simulink model "SimDraft1"  (R2024a)
settings: Solver=VariableStepAuto  StartTime=0.0  StopTime=2  RelTol=1e-3
model workspace (MAT data in the model file):
  CanaryCarrierFrequency = 20000
  CanaryDataRate = 100
  SampleRate = 44100
undefined symbols (not defined in the file or in its folder): azelaxes, fdesignblkfcn, gcbh, physconst
libraries: audiosources x2, dspfdesign x2, commseqgen3 x2, dspfiltersrcs x1, dspmlti4 x1, commanapbnd3 x1, dsparch4 x1, commdigbbndam3 x1, phasedenvlib x1
settings Model: Creator=calum  LastModifiedBy=calum

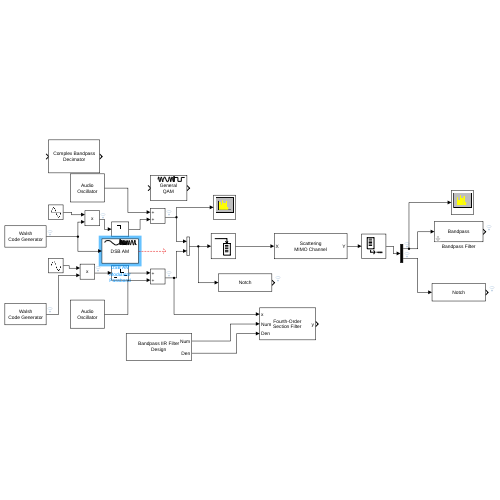
[thumbnail: Simulink's stored preview of the top-level diagram]
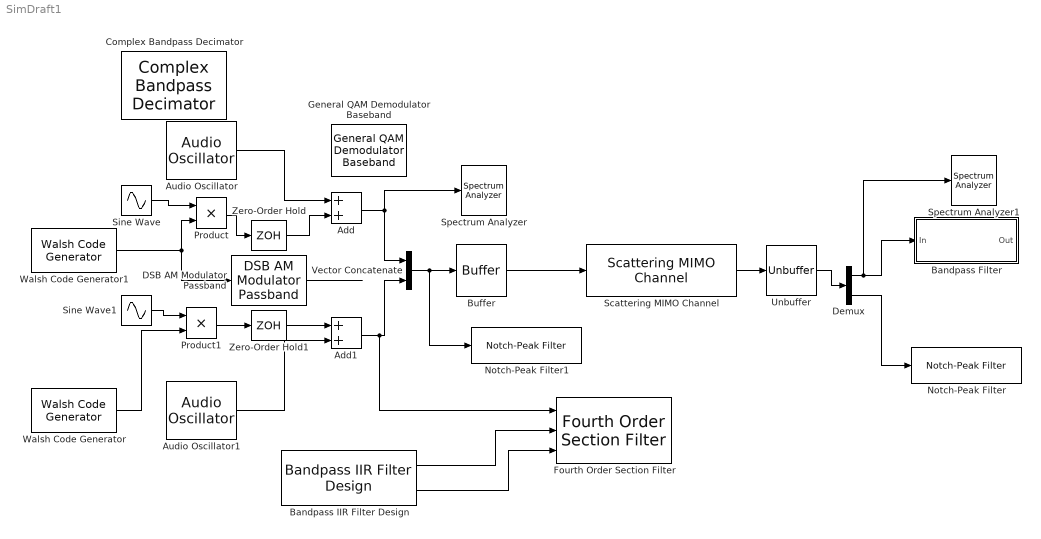
== system SimDraft1 ==
  Add : Sum
  Add1 : Sum
  Audio Oscillator : audiosources/Audio Oscillator  FrequencyPort=off  Frequency=200  AmplitudePort=off  Amplitude=1  DCOffsetPort=off  DCOffset=0  PhaseOffset=0  WidthPort=off  Width=1  DutyCyclePort=off  DutyCycle=0.5  SampsPerFrame=1  Fs=SampleRate  OutputDataType=double  SimulateUsing=Code generation
      settings: SignalType=sine
  Audio Oscillator1 : audiosources/Audio Oscillator  FrequencyPort=off  Frequency=500  AmplitudePort=off  Amplitude=1  DCOffsetPort=off  DCOffset=0  PhaseOffset=0  WidthPort=off  Width=1  DutyCyclePort=off  DutyCycle=0.5  SampsPerFrame=1  Fs=SampleRate  OutputDataType=double  SimulateUsing=Code generation
      settings: SignalType=sine
  Bandpass Filter : Subsystem  DialogController=fdesignblkfcn  InitFcn=fdesignblkfcn(gcbh, {'InitFcn'});  mask(Bandpass Filter){}
      mask help: dsp:DSPFilterDesignBlockDialog:BandpassFdesign_MaskDesc
      settings: CopyFcn=fdesignblkfcn(gcbh, {'CopyFcn'});
      mask Help: helpview(mapfilelocation('dsp'), 'dspbandpassfilter');
      mask Display: disp('Bandpass');
  Bandpass IIR Filter Design : dspfiltersrcs/Bandpass IIR Filter Design  SmoothParameters=off  SmoothingFactor=0.6  DesignMethod=Butterworth  FilterOrderPort=off  FilterOrder=6  MaxOrder=10  F3dB1Port=off  F3dB1=(CanaryCarrierFrequency-CanaryDataRate)/SampleRate/2  F3dB2Port=off  F3dB2=(CanaryCarrierFrequency+CanaryDataRate)/SampleRate/2  ApassPort=off  Apass=1  AstopPort=off  Astop=60  CascadeSectionsForm=Fourth-order sections  HasScaleValues=off  OutputDataType=double  SampleTime=-1  SimulateUsing=Interpreted execution
  Buffer : Buffer  OutputFrames=off
  Complex Bandpass Decimator : dspmlti4/Complex Bandpass Decimator  Specification=Bandwidth  DecimationFactor=2  Bandwidth=CanaryDataRate  CenterFrequencyPort=off  CenterFrequency=CanaryCarrierFrequency  StopbandAttenuation=80  PassbandRipple=1  TransitionWidth=40  MinimizeComplexCoefficients=on  MixToBaseband=on  InheritSampleRate=off  SampleRate=SampleRate  AllowArbitraryInputLength=off  SimulateUsing=Interpreted execution
  DSB AM Modulator Passband : commanapbnd3/DSB AM Modulator Passband  Fc=CanaryCarrierFrequency  Ph=0  Offset=1
  Demux : Demux  Outputs=2
  Fourth Order Section Filter : dsparch4/Fourth Order Section Filter  CoefficientSource=Input ports  Numerator=[0.07795634 0 -0.15591268 0 0.07795634; 0.06188520 0 -0.12377039 0 0.06188520]  Denominator=[1 0 1.32091343 0 0.63273879; 1 0 1.04859957 0 0.29614035]  FilterObject=dsp.FourthOrderSectionFilter  SimulateUsing=Code generation
  General QAM Demodulator Baseband : commdigbbndam3/General QAM Demodulator Baseband  SigCon=[exp(2*pi*1i*[0:7]/8)]  OutType=Integer  DecType=Hard decision  VarSource=Dialog  Variance=1  outDtypeBit=Inherit via internal rule  outDtype=Inherit via internal rule  roundingMode=Floor  overflowMode=Wrap  OvFlMode=off  OvFlModeLastStrValue=off  sigConstWordLen=16  sigConstDataTypeStr=Inherit: Same word length as input  sigConstLastDataTypeStr=Inherit: Same word length as input  accum1WordLen=32  accum1FracLen=30  prodInWordLen=32  prodInFracLen=30  prodInDataTypeStr=Inherit: Same as accumulator 1  prodInLastDataTypeStr=Inherit: Same as accumulator 1  prodOutWordLen=32  prodOutFracLen=30  accum2WordLen=32  accum2FracLen=30  accum3WordLen=32  accum3FracLen=30  nsiWordLen=32  nsiFracLen=30  nsiDataTypeStr=Inherit: Same as accumulator 3  nsiLastDataTypeStr=Inherit: Same as accumulator 3  invn0WordLen=16  invn0FracLen=8  invn0DataTypeStr=Inherit: Same word length as input  invn0LastDataTypeStr=Inherit: Same word length as input  outputWordLen=32  outputFracLen=30
  Notch-Peak Filter : dspfdesign/Notch-Peak Filter  Specification=Bandwidth and center frequency  BandwidthPort=off  Bandwidth=200  QualityFactorPort=off  QualityFactor=5  CenterFrequencyPort=off  CenterFrequency=20000  BandwidthCoefficientPort=off  BandwidthCoefficient=0.72654  CenterFrequencyCoefficientPort=off  CenterFrequencyCoefficient=0  Output=Notch  SampleRateMode=Specify on dialog  SampleRate=44100  SimulateUsing=Code generation
  Notch-Peak Filter1 : dspfdesign/Notch-Peak Filter  Specification=Bandwidth and center frequency  BandwidthPort=off  Bandwidth=200  QualityFactorPort=off  QualityFactor=5  CenterFrequencyPort=off  CenterFrequency=CanaryCarrierFrequency  BandwidthCoefficientPort=off  BandwidthCoefficient=0.72654  CenterFrequencyCoefficientPort=off  CenterFrequencyCoefficient=0  Output=Notch  SampleRateMode=Specify on dialog  SampleRate=SampleRate  SimulateUsing=Code generation
  Product : Product
  Product1 : Product
  Scattering MIMO Channel : phasedenvlib/Scattering MIMO Channel  PropagationSpeed=300  CarrierFrequency=CanaryCarrierFrequency  Polarization=None  SpecifyAtmosphere=off  Temperature=15  DryAirPressure=101325  WaterVapourDensity=7.5  LiquidWaterDensity=0  RainRate=0  SampleRateFromInputCheckbox=on  SampleRate=1e6  SimulateDirectPath=on  MaximumDelaySource=Property  MaximumDelay=2  ChannelResponseOutputPort=off  SimulateUsing=Code generation  TransmitArray=phased.ULA(Element=phased.OmnidirectionalMicrophoneElement())  ReceiveArray=phased.ULA(Element=phased.OmnidirectionalMicrophoneElement())  TransmitArrayMotionSource=Property  TransmitArrayPosition=[ 0; 0; 0 ]  TransmitArrayOrientationAxes=eye( 3 )  ReceiveArrayMotionSource=Property  ReceiveArrayPosition=[ 10; 0; 0 ]  ReceiveArrayOrientationAxes=azelaxes( 180, 0 )  ScattererSpecificationSource=Auto  NumScatterers=0  ScattererPositionBoundary=[ 0, 1000 ]  ScattererPosition=[ physconst( 'LightSpeed' )*5e-6; 0; 0 ]  ScattererCoefficient=1  ScatteringMatrix=eye( 2 )  ScattererOrientationAxes=eye( 3 )  SeedSource=Auto  Seed=0
  Sine Wave : Sin  Frequency=2*pi*CanaryCarrierFrequency  SampleTime=0
  Sine Wave1 : Sin  Frequency=2*pi*CanaryCarrierFrequency  SampleTime=0
  Spectrum Analyzer : SpectrumAnalyzer  SampleRateSource=Property  SampleRate=44.1e3  PlotAsTwoSidedSpectrum=off  FrequencyScale=Log  FrequencySpan=Start and stop frequencies  StartFrequency=20  StopFrequency=20e3
  Spectrum Analyzer1 : SpectrumAnalyzer  SampleRateSource=Property  SampleRate=44.1e3  PlotAsTwoSidedSpectrum=off  FrequencyScale=Log  FrequencySpan=Start and stop frequencies  StartFrequency=20  StopFrequency=20e3
  Unbuffer : Unbuffer
  Vector Concatenate : Concatenate  Mode=Multidimensional array  ConcatenateDimension=2
  Walsh Code Generator : commseqgen3/Walsh Code Generator  Length=16  Index=8  SampleTime=1/CanaryDataRate  SamplesPerFrame=1  OutputDataType=double  SimulateUsing=Code generation
  Walsh Code Generator1 : commseqgen3/Walsh Code Generator  Length=16  Index=8  SampleTime=1/CanaryDataRate  SamplesPerFrame=1  OutputDataType=double  SimulateUsing=Code generation
  Zero-Order Hold : ZeroOrderHold  SampleTime=1/SampleRate
  Zero-Order Hold1 : ZeroOrderHold  SampleTime=1/SampleRate
  wires:
  Vector Concatenate/1 -> Notch-Peak Filter1/1, Buffer/1
  Sine Wave/1 -> Product/1
  Sine Wave1/1 -> Product1/1
  Walsh Code Generator/1 -> Product1/2
  Product/1 -> Zero-Order Hold/1
  Audio Oscillator/1 -> Add/1
  Add/1 -> Vector Concatenate/1, Spectrum Analyzer/1
  Add1/1 -> Fourth Order Section Filter/1, Vector Concatenate/2
  Product1/1 -> Zero-Order Hold1/1
  Audio Oscillator1/1 -> Add1/2
  Scattering MIMO Channel/1 -> Unbuffer/1
  Zero-Order Hold/1 -> Add/2
  Zero-Order Hold1/1 -> Add1/1
  Buffer/1 -> Scattering MIMO Channel/1
  Unbuffer/1 -> Demux/1
  Demux/1 -> Spectrum Analyzer1/1, Bandpass Filter/1(In)
  Demux/2 -> Notch-Peak Filter/1
  DSB AM Modulator Passband/1 -> ?
  Walsh Code Generator1/1 -> Product/2, DSB AM Modulator Passband/1
  Bandpass IIR Filter Design/1 -> Fourth Order Section Filter/2
  Bandpass IIR Filter Design/2 -> Fourth Order Section Filter/3

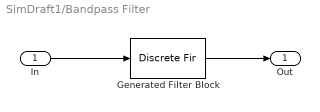
== system SimDraft1/Bandpass Filter ==
  In : Inport
  Generated Filter Block : DiscreteFir  Tag=BlockMethodSubSystem  Coefficients=[0.00111455429792117256 -0.001830035238418466 0.00300586016208201096 -0.00432566826021033284 0.00559141715902218735 -0.00655844264883879632 0.00698597455582325097 -0.00669792865803245027 0.00564097851855352439 -0.00392739220773750258 0.0018439081478687086 0.000183050467559543739 -0.00166267787164066372 0.00214482380872847017 -0.00133589152998281335 -0.000802556524375712399 0.00400181589900176771 -0.00770034250859667063 0.0111301921197185655 -0.0134666689276723567 0.0140151971415618248 -0.0123943490952151403 0.00866904196237028302 -0.0033952251265152722 -0.00244666560955103529 0.00762982155398304884 -0.0109442372674948413 0.011493705177076291 -0.00896093526897952242 0.00377504342804718673 0.00286978379325457389 -0.00916793411761730737 0.0130154315465422221 -0.012432410449106035 0.00601561171461237332 0.00667329787022853671 -0.0248730983576116171 0.0466063354776198452 -0.0689037461289037784 0.0882447869312457805 -0.101143456889725328 0.104774330301750651 -0.0975192982084671645 0.0793255491042365035 -0.0517983849248481176 0.0180020369893912902 0.0180020369893912902 -0.0517983849248481176 0.0793255491042365035 -0.0975192982084671645 0.104774330301750651 -0.101143456889725328 0.0882447869312457805 -0.0689037461289037784 0.0466063354776198452 -0.0248730983576116171 0.00667329787022853671 0.00601561171461237332 -0.012432410449106035 0.0130154315465422221 -0.00916793411761730737 0.00286978379325457389 0.00377504342804718673 -0.00896093526897952242 0.011493705177076291 -0.0109442372674948413 0.00762982155398304884 -0.00244666560955103529 -0.0033952251265152722 0.00866904196237028302 -0.0123943490952151403 0.0140151971415618248 -0.0134666689276723567 0.0111301921197185655 -0.00770034250859667063 0.00400181589900176771 -0.000802556524375712399 -0.00133589152998281335 0.00214482380872847017 -0.00166267787164066372 0.000183050467559543739 0.0018439081478687086 -0.00392739220773750258 0.00564097851855352439 -0.00669792865803245027 0.00698597455582325097 -0.00655844264883879632 0.00559141715902218735 -0.00432566826021033284 0.00300586016208201096 -0.001830035238418466 0.00111455429792117256]  InputProcessing=Columns as channels (frame based)
  Out : Outport  VectorParamsAs1DForOutWhenUnconnected=off
  wires:
  In/1 -> Generated Filter Block/1
  Generated Filter Block/1 -> Out/1
